simulink model "BESS_Harness"  (R2025b)
settings: Solver=VariableStepAuto  StartTime=0.0  StopTime=5  RelTol=1e-3
PostLoadFcn:
  | BESSParam
values from neighbouring files (symbols this model uses):
  bessVoltage = 1500    [BESSGFLParam.m]    (also in BESSGFMParam.m)
  gflInverter = struct    [BESSGFLParam.m]
  gfmInverter = struct    [BESSGFMParam.m]
  Ts = 5E-5    (= 5e-05)    [BESSGFLParam.m]    (also in BESSGFMParam.m; WindFarmParam.m)
undefined symbols (not defined in the file or in its folder): bessSystem, DiscIntNeverNeededParam, solar
libraries: eeGeneralControl x26, nesl_utility x26, ee_lib x16, simulink x12, fl_lib x10, eeTransforms x7, nesl_utility_internal x4, slpidlib x2, batteryecm_lib x2, simulink_extras x1, eePowerMeasurement x1, eePwmGenerator x1
(part 3 of 4)

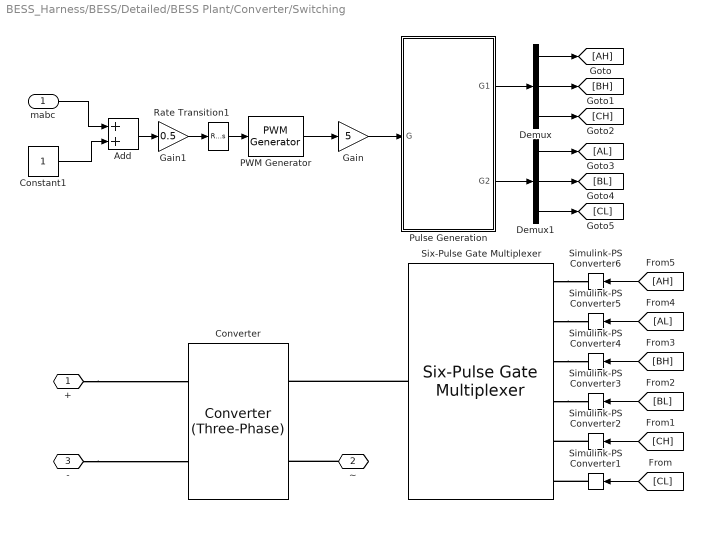
== system BESS_Harness/BESS/Detailed/BESS Plant/Converter/Switching ==
  mabc : Inport
  Add : Sum
  Constant1 : Constant
  Converter : ee_lib/Semiconductors & Converters/Converters/Converter (Three-Phase)  port_option=ee.enum.threePhasePort.composite  fidelity_option=ee.enum.converters.fidelity.detailed  device_type=ee.enum.converters.switchingdevice.ideal  showThermalPort=false  K=0  Vth=1 V  Vgt=1 V  Vgt_off=-1 V  Ih=1 A  Vf=0.8 V  Ron=0.001 Ohm  Rds=0.001 Ohm  Goff=1e-6 1/Ohm  Eon_scalar=22.86e-3 J  Eoff_scalar=17.14e-3 J  Eoff_natural_commutation=10e-3 J  Voff=300 V  Iout_scalar=600 A  onCurrentMeasDelay=0 s  useCurrentFromPreviousCycle=false  useVoltageFromPreviousCycle=false  diode_param=ee.enum.converters.protectiondiode.nodynamics  diode_Vf=0.01 V  diode_Ron=0.0001 Ohm  diode_Goff=1e-5 1/Ohm  diode_C=50 nF  diode_iRM=-235 A  diode_iF=300 A  diode_idot=-50 A/us  diode_trr_param=ee.enum.converters.diodetrr.trr_factor  diode_trr_factor=3  diode_trr=15 us  diode_Qrr=1500 s*uA  diode_rec_loss_model=ee.enum.diode.reverseRecoveryModel.fixed  diode_ErecVal=0 J  diode_scaleWithIandV=false  diode_ErecMat=zeros(2, 3) J  diode_TjrecVec=[298.15, 398.15] K  diode_IfrecVec=[.1, 1, 10] A  diode_IrecVal=10 A  diode_VrecVal=10 V  diode_tFilter=1 / 1000 / 100 s  thermal_network_parameterization=ee.enum.thermalNetworkTopology.external  Rth=[.08, .5] K/W  Rth_Cauer=[.08, .1, .5] K/W  Rth_Foster=[.08, .14, .22, .16] K/W  thermal_mass_parameterization=ee.enum.thermalNetwork.timeconstant  thermal_mass=[.01, .5] J/K  thermal_mass_Cauer=[.01, .1, .5] J/K  thermal_mass_Foster=[.001, .005, .05, .5] J/K  thermal_time_constant=[.001, .2] s  thermal_time_constant_Cauer=[.001, .1, .2] s  thermal_time_constant_Foster=[7e-05, .0007, .01, .08] s  thermal_mass_initial_temperatures=[25, 25] degC  thermal_mass_initial_temperatures_Cauer=[25, 25, 25] degC  junction_thermal_mass=0.01 J/K  Tvec_initial_Foster=[25, 25, 25, 25] degC  snubber_type=ee.enum.converters.snubber.exclude  Cs=1e-7 F  Rs=0.1 Ohm  Vce_loss=[0, 150, 300] V
  Demux : Demux  Outputs=3
  Demux1 : Demux  Outputs=3
  Gain : Gain  Gain=5
  Gain1 : Gain  Gain=0.5
  PWM Generator : eePwmGenerator/PWM Generator  CarrCount=Up  Tper=1/(fSw*1000)  Tdelay=0  Ts=1/(10*fSw*1000)
  Pulse Generation : Subsystem
  Rate Transition1 : RateTransition  OutPortSampleTime=1/(10*fSw*1000)
  Simulink-PS Converter{1..6} (6 alike) : nesl_utility/Simulink-PS Converter  PhysicalDomain=network_engine_domain  SubClassName=ps_input  LeftPortType=input  RightPortType=output  PseudoPeriodic=off  Frequencies=[]  NoiseDistribution=none  NoiseParameters=[]  Unit=1  AffineConversion=off  FilteringAndDerivatives=provide  SimscapeFilterOrder=1  InputFilterTimeConstant=0.001  UdotUserProvided=0
  Six-Pulse Gate Multiplexer : ee_lib/Semiconductors & Converters/Converters/Six-Pulse Gate Multiplexer  port_option=ee.enum.controlport.ps
  + : PMIOPort  Side=Left
  ~ : PMIOPort  Port=2  Side=Right
  - : PMIOPort  Port=3  Side=Left
  wires:
  Demux1/1 -> [AL]
  [BL] -> Simulink-PS Converter3/1
  [AH] -> Simulink-PS Converter6/1
  Demux1/3 -> [CL]
  Gain1/1 -> Rate Transition1/1
  Demux/3 -> [CH]
  Demux/2 -> [BH]
  [CL] -> Simulink-PS Converter1/1
  Constant1/1 -> Add/2
  Add/1 -> Gain1/1
  Gain/1 -> Pulse Generation/1(G)
  PWM Generator/1 -> Gain/1
  mabc/1 -> Add/1
  [CH] -> Simulink-PS Converter2/1
  [AL] -> Simulink-PS Converter5/1
  Demux1/2 -> [BL]
  Demux/1 -> [AH]
  Rate Transition1/1 -> PWM Generator/1
  Pulse Generation/2(G2) -> Demux1/1
  Pulse Generation/1(G1) -> Demux/1
  [BH] -> Simulink-PS Converter4/1
  connections:
  ~/RConn1 -- Converter/LConn2
  Six-Pulse Gate Multiplexer/LConn2 -- Simulink-PS Converter5/RConn1
  Simulink-PS Converter2/RConn1 -- Six-Pulse Gate Multiplexer/LConn5
  Simulink-PS Converter1/RConn1 -- Six-Pulse Gate Multiplexer/LConn6
  Six-Pulse Gate Multiplexer/LConn3 -- Simulink-PS Converter4/RConn1
  Six-Pulse Gate Multiplexer/RConn1 -- Converter/LConn1
  Six-Pulse Gate Multiplexer/LConn1 -- Simulink-PS Converter6/RConn1
  Six-Pulse Gate Multiplexer/LConn4 -- Simulink-PS Converter3/RConn1
  +/RConn1 -- Converter/RConn1
  -/RConn1 -- Converter/RConn2

== system BESS_Harness/BESS/Detailed/Filter & Measurements/PLL & Measurements/Measurement1 ==
  u : Inport
  Lead-Lag (Discrete or Continuous) : eeGeneralControl/Lead-Lag (Discrete or Continuous)  T1=0  T2=1e-3  B=inf  A=-inf  init_option=Inherited from block input  x0=0  Ts=Ts
  Vg : Outport
  wires:
  u/1 -> Lead-Lag (Discrete or Continuous)/1
  Lead-Lag (Discrete or Continuous)/1 -> Vg/1

== system BESS_Harness/BESS/Detailed/Filter & Measurements/PLL & Measurements/Measurement2 ==
  u : Inport
  Lead-Lag (Discrete or Continuous) : eeGeneralControl/Lead-Lag (Discrete or Continuous)  T1=0  T2=1e-3  B=inf  A=-inf  init_option=Inherited from block input  x0=0  Ts=Ts
  Vg : Outport
  wires:
  u/1 -> Lead-Lag (Discrete or Continuous)/1
  Lead-Lag (Discrete or Continuous)/1 -> Vg/1

== system BESS_Harness/BESS/Detailed/Filter & Measurements/PLL & Measurements/Subsystem ==
  Vabc : Inport
  Iabc : Inport  Port=2
  Demux : Demux  Outputs=3
  Demux1 : Demux  Outputs=3
  Park Transform : eeTransforms/Park Transform  AxisAlignment=Q-axis  PowerInvariant=off
  Park Transform1 : eeTransforms/Park Transform  AxisAlignment=Q-axis  PowerInvariant=off
  Scope : Scope  NumInputPorts=2
      settings: ActiveDisplayYMinimum=0.95416  ActiveDisplayYMaximum=1.02793  DataLoggingVariableName=ScopeData5
  Scope1 : Scope  NumInputPorts=2
      settings: ActiveDisplayYMinimum=-2.7903298017751648  ActiveDisplayYMaximum=-1.7770998587100291  DataLoggingVariableName=ScopeData10
  "Sinusoidal Measurement (PLL, Three-Phase)" : eeSinusoidalMeasurementV2/Sinusoidal Measurement (PLL, Three-Phase)  InputFilter=on  InputNormalization=off  Kp_LF=40  Ki_LF=1000  F0=frequency  Theta0=0  Ts=Ts
  Terminator : Terminator
  Terminator1 : Terminator
  mag : Outport
  freq : Outport  Port=2
  angle : Outport  Port=3
  Vd : Outport  Port=4
  Vq : Outport  Port=5
  Id1 : Outport  Port=6
  Iq1 : Outport  Port=7
  wires:
  Iabc/1 -> Park Transform1/1
  Demux1/3 -> Terminator1/1
  Demux1/2 -> Scope1/2, Iq1/1
  Demux1/1 -> Scope1/1, Id1/1
  Park Transform1/1 -> Demux1/1
  "Sinusoidal Measurement (PLL, Three-Phase)"/3 -> mag/1
  "Sinusoidal Measurement (PLL, Three-Phase)"/1 -> freq/1
  "Sinusoidal Measurement (PLL, Three-Phase)"/2 -> Park Transform/2, Park Transform1/2, angle/1
  Demux/2 -> Vq/1, Scope/2
  Demux/1 -> Vd/1, Scope/1
  Park Transform/1 -> Demux/1
  Vabc/1 -> "Sinusoidal Measurement (PLL, Three-Phase)"/1, Park Transform/1
  Demux/3 -> Terminator/1

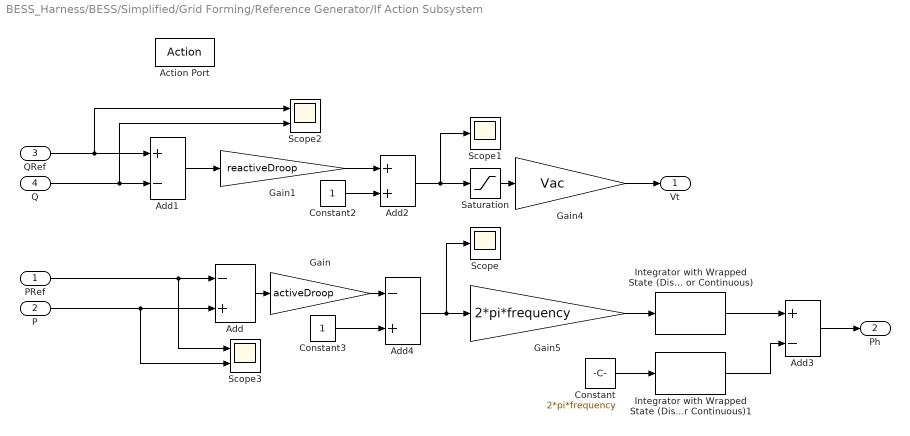
== system BESS_Harness/BESS/Simplified/Grid Forming/Reference Generator/If Action Subsystem ==
  PRef : Inport
  P : Inport  Port=2
  QRef : Inport  Port=3
  Q : Inport  Port=4
  Action Port : ActionPort  ActionPortLabel=if(u1 > 0)
  Add : Sum  Inputs=-+
  Add1 : Sum  Inputs=+-
  Add2 : Sum
  Add3 : Sum  Inputs=+-
  Add4 : Sum  Inputs=-+
  Constant : Constant  Value=2*pi*frequency  SampleTime=-1
  Constant2 : Constant
  Constant3 : Constant
  Gain : Gain  Gain=activeDroop
  Gain1 : Gain  Gain=reactiveDroop
  Gain4 : Gain  Gain=Vac
  Gain5 : Gain  Gain=2*pi*frequency
  Integrator with Wrapped State (Discrete or Continuous) : eeGeneralControl/Integrator with Wrapped State (Discrete or Continuous)  LabelModeActiveChoice=Discrete  WrappedStateUpperValue=2*pi  WrappedStateLowerValue=0  x0=0  Ts=-1
  Integrator with Wrapped State (Discrete or Continuous)1 : eeGeneralControl/Integrator with Wrapped State (Discrete or Continuous)  LabelModeActiveChoice=Discrete  WrappedStateUpperValue=2*pi  WrappedStateLowerValue=0  x0=0  Ts=-1
  Saturation : Saturate  UpperLimit=1.1  LowerLimit=0.9
  Scope : Scope
      settings: ActiveDisplayYMinimum=-1  ActiveDisplayYMaximum=1  DataLoggingVariableName=ScopeData2
  Scope1 : Scope
      settings: ActiveDisplayYMinimum=-1  ActiveDisplayYMaximum=1  DataLoggingVariableName=ScopeData3
  Scope2 : Scope  NumInputPorts=2
      settings: ActiveDisplayYMinimum=-1  ActiveDisplayYMaximum=1
  Scope3 : Scope  NumInputPorts=2
      settings: ActiveDisplayYMinimum=-1  ActiveDisplayYMaximum=1  DataLoggingVariableName=ScopeData2
  Vt : Outport
  Ph : Outport  Port=2
  wires:
  Add4/1 -> Scope/1, Gain5/1
  Gain/1 -> Add4/1
  Add1/1 -> Gain1/1
  Add2/1 -> Scope1/1, Saturation/1
  Gain5/1 -> Integrator with Wrapped State (Discrete or Continuous)/1
  Constant3/1 -> Add4/2
  Integrator with Wrapped State (Discrete or Continuous)/1 -> Add3/1
  Constant2/1 -> Add2/2
  Gain1/1 -> Add2/1
  Gain4/1 -> Vt/1
  QRef/1 -> Add1/1, Scope2/1
  Saturation/1 -> Gain4/1
  Add/1 -> Gain/1
  PRef/1 -> Add/1, Scope3/1
  Add3/1 -> Ph/1
  Constant/1 -> Integrator with Wrapped State (Discrete or Continuous)1/1
  Integrator with Wrapped State (Discrete or Continuous)1/1 -> Add3/2
  P/1 -> Add/2, Scope3/2
  Q/1 -> Add1/2, Scope2/2

== system BESS_Harness/BESS/Simplified/Grid Forming/Reference Generator/If Action Subsystem1 ==
  PRef : Inport
  P : Inport  Port=2
  VRef : Inport  Port=3
  V : Inport  Port=4
  Action Port : ActionPort  ActionPortLabel=else
  Add : Sum  Inputs=+-
  Add1 : Sum  Inputs=+-
  Add2 : Sum
  Add3 : Sum  Inputs=+-
  Add4 : Sum  Inputs=-+
  Constant2 : Constant
  Constant3 : Constant
  Constant4 : Constant  Value=0
  Gain : Gain  Gain=reactiveDroop
  Gain1 : Gain  Gain=activeDroop
  Gain4 : Gain  Gain=systemVoltage
  Gain5 : Gain  Gain=2*pi*systemFrequency
  Integrator with Wrapped State (Discrete or Continuous) : eeGeneralControl/Integrator with Wrapped State (Discrete or Continuous)  LabelModeActiveChoice=Discrete  WrappedStateUpperValue=2*pi  WrappedStateLowerValue=0  x0=0  Ts=-1
  Saturation : Saturate  UpperLimit=1.1  LowerLimit=0.9
  Vt : Outport
  Ph : Outport  Port=2
  wires:
  Add/1 -> Gain/1
  Constant4/1 -> Add3/2
  Add4/1 -> Gain5/1
  Gain/1 -> Add4/1
  Add1/1 -> Gain1/1
  Add2/1 -> Saturation/1
  Gain5/1 -> Integrator with Wrapped State (Discrete or Continuous)/1
  Constant3/1 -> Add4/2
  Integrator with Wrapped State (Discrete or Continuous)/1 -> Add3/1
  Constant2/1 -> Add2/2
  Gain1/1 -> Add2/1
  V/1 -> Add/2
  Gain4/1 -> Vt/1
  P/1 -> Add1/2
  VRef/1 -> Add/1
  PRef/1 -> Add1/1
  Add3/1 -> Ph/1
  Saturation/1 -> Gain4/1

== system BESS_Harness/BESS/Detailed/BESS Controller/Grid Following/Reference Current/Current limits ==
  Imax : Inport
  iqref : Inport  Port=2
  idref : Inport  Port=3
  Constant8 : Constant  Value=0
  Constant9 : Constant  Value=0
  Scope : Scope
      settings: ActiveDisplayYMinimum=-0.14399  ActiveDisplayYMaximum=1.29587  DataLoggingVariableName=ScopeData3
  Scope1 : Scope
      settings: ActiveDisplayYMinimum=-0.13655  ActiveDisplayYMaximum=1.22893  DataLoggingVariableName=ScopeData4
  Sqrt : Sqrt
  Sqrt1 : Sqrt
  Square{1..4} (4 alike) : Math  Operator=square
  Step2 : Step  Time=0.01  SampleTime=Ts
  Step3 : Step  Time=0.01  SampleTime=Ts
  Sum6 : Sum  Inputs=|+-
  Sum9 : Sum  Inputs=|+-
  Switch1 : Switch  Threshold=.01  SaturateOnIntegerOverflow=off  InputSameDT=off
  Switch2 : Switch  Threshold=.01  SaturateOnIntegerOverflow=off  InputSameDT=off
  iubq : Outport
  iubd : Outport  Port=2
  wires:
  idref/1 -> Square4/1
  Sqrt1/1 -> iubq/1, Scope1/1
  Imax/1 -> Square1/1, Square3/1
  Sqrt/1 -> iubd/1, Scope/1
  Constant9/1 -> Switch2/3
  Square4/1 -> Sum9/2
  Constant8/1 -> Switch1/3
  Square2/1 -> Sum6/2
  Sum6/1 -> Switch1/1
  Square3/1 -> Sum9/1
  iqref/1 -> Square2/1
  Switch1/1 -> Sqrt/1
  Square1/1 -> Sum6/1
  Switch2/1 -> Sqrt1/1
  Step2/1 -> Switch1/2
  Step3/1 -> Switch2/2
  Sum9/1 -> Switch2/1

== system BESS_Harness/BESS/Detailed/BESS Controller/Grid Following/Reference Current/Refernce id generation ==
  V_mag : Inport
  del f : Inport  Port=2
  ubid : Inport  Port=3
  PRef : Inport  Port=4
  Divide : Product  Inputs=/*
  Gain6 : Gain  Gain=-1
  P/Q Priority : Switch  Criteria=u2 ~= 0  SaturateOnIntegerOverflow=off  InputSameDT=off
  Priority Mode : Constant  Value=P-2
  Saturation Dynamic2 : simulink/Discontinuities/Saturation Dynamic  OutMin=[]  OutMax=[]  OutDataTypeStr=Inherit: Same as second input  OutDataType=fixdt(1, 16)  OutScaling=2^-10  DoSatur=off
  Saturation1 : Saturate  UpperLimit=Imax  LowerLimit=-Imax
  Scope : Scope
      settings: ActiveDisplayYMinimum=-1  ActiveDisplayYMaximum=1
  Scope1 : Scope
      settings: ActiveDisplayYMinimum=-0.68622  ActiveDisplayYMaximum=0.07625  DataLoggingVariableName=ScopeData2
  Sum : Sum  Inputs=|++
  droop m_p : Gain  Gain=mp/MVA
  ubid1 : InportShadow  Port=3
  id_ref : Outport
  wires:
  del f/1 -> droop m_p/1
  Divide/1 -> Saturation Dynamic2/2, Saturation1/1
  V_mag/1 -> Divide/1
  P/Q Priority/1 -> id_ref/1, Scope/1
  ubid1/1 -> Gain6/1
  Saturation1/1 -> P/Q Priority/1
  Priority Mode/1 -> P/Q Priority/2
  PRef/1 -> Sum/2
  Saturation Dynamic2/1 -> P/Q Priority/3, Scope1/1
  Gain6/1 -> Saturation Dynamic2/3
  ubid/1 -> Saturation Dynamic2/1
  Sum/1 -> Divide/2
  droop m_p/1 -> Sum/1

== system BESS_Harness/BESS/Detailed/BESS Controller/Grid Following/Reference Current/Refernce iq generation ==
  ubiq : Inport
  V_ref : Inport  Port=2
  V_mag : Inport  Port=3
  LVRT_iq : Inport  Port=4
  Q_ref : Inport  Port=5
  Divide1 : Product  Inputs=*/
  Gain : Gain  Gain=-1
  Gain1 : Gain  Gain=-1
  Gain7 : Gain  Gain=-1
  LVRT Priority : Switch  Threshold=.9  SaturateOnIntegerOverflow=off  InputSameDT=off
  P/Q Priority : Switch  Criteria=u2 ~= 0  SaturateOnIntegerOverflow=off  InputSameDT=off
  Priority Mode : Constant  Value=P-2
  Saturation Dynamic : simulink/Discontinuities/Saturation Dynamic  OutMin=[]  OutMax=[]  OutDataTypeStr=Inherit: Same as second input  OutDataType=fixdt(1, 16)  OutScaling=2^-10  DoSatur=off
  Saturation2 : Saturate  UpperLimit=1  LowerLimit=-1
  Saturation3 : Saturate  UpperLimit=Imax  LowerLimit=-Imax
  Sum : Sum  Inputs=|++
  Sum1 : Sum  Inputs=|-+
  droop m_v : Gain  Gain=mv
  ubiq1 : InportShadow
  iq_ref : Outport
  wires:
  Gain/1 -> iq_ref/1
  V_mag/1 -> Sum1/2, Divide1/2, LVRT Priority/2
  Q_ref/1 -> Sum/1
  Sum/1 -> Divide1/1
  droop m_v/1 -> Sum/2
  ubiq1/1 -> Gain7/1
  LVRT_iq/1 -> Saturation2/1
  V_ref/1 -> Sum1/1
  Gain7/1 -> Saturation Dynamic/3
  Saturation Dynamic/1 -> P/Q Priority/1
  Divide1/1 -> Saturation3/1, Saturation Dynamic/2
  Priority Mode/1 -> P/Q Priority/2
  Saturation3/1 -> P/Q Priority/3
  Saturation2/1 -> Gain1/1
  ubiq/1 -> Saturation Dynamic/1
  Gain1/1 -> LVRT Priority/3
  P/Q Priority/1 -> LVRT Priority/1
  Sum1/1 -> droop m_v/1
  LVRT Priority/1 -> Gain/1

== system BESS_Harness/BESS/Detailed/BESS Controller/Grid Forming/Current Limiting/CurrentLimitingMethod ==
  Igd : Inport
  Igq : Inport  Port=2
  currentLimitAndVirtual : Subsystem  VariantControl=both
  currentSaturation : Subsystem  VariantControl=ctSat
  virtualImpedance : Subsystem  VariantControl=virimp
  delVd : Outport
  delVq : Outport  Port=2
  Idmax : Outport  Port=3
  Iqmax : Outport  Port=4

== system BESS_Harness/BESS/Detailed/BESS Controller/Grid Forming/Grid Voltage Reactive Power Support/Modifying Active Power Reference ==
  PrefInput : Inport
  Vd : Inport  Port=2
  Igd : Inport  Port=3
  Igq : Inport  Port=4
  AND : Logic  IconShape=distinctive  AllPortsSameDT=off  OutDataTypeStr=boolean
  Abs : Abs  SaturateOnIntegerOverflow=off
  Compare To Constant : simulink/Logic and Bit Operations/Compare To Constant  relop=>=  const=0.95  OutDataTypeStr=boolean
  Computing New Active Power Ref : Subsystem
  Math Function1 : Math  Operator=hypot
  Power Sign : Signum
  Product : Product
  Relay : Relay  OnSwitchValue=40%maxVICurrentLimit*0.96  OffSwitchValue=1
  Scope : Scope
  Scope1 : Scope
  Scope2 : Scope
  Switch : Switch  Criteria=u2 > Threshold  SaturateOnIntegerOverflow=off  InputSameDT=off
  Pref : Outport
  wires:
  Compare To Constant/1 -> AND/1
  AND/1 -> Switch/2
  Relay/1 -> AND/2, Scope1/1
  Product/1 -> Pref/1
  Power Sign/1 -> Product/2
  Abs/1 -> Product/1
  Switch/1 -> Abs/1
  Igq/1 -> Math Function1/1, Computing New Active Power Ref/1(Iq)
  Igd/1 -> Math Function1/2
  PrefInput/1 -> Switch/3, Power Sign/1
  Vd/1 -> Compare To Constant/1, Computing New Active Power Ref/2(Vd)
  Math Function1/1 -> Relay/1, Scope2/1  "Is"
  Computing New Active Power Ref/1(Pref) -> Scope/1, Switch/1

== system BESS_Harness/BESS/Detailed/BESS Controller/Grid Forming/Grid Voltage Reactive Power Support/Modifying Reactive Power Reference ==
  Vgd : Inport
  Vgq : Inport  Port=2
  Qref : Inport  Port=3
  Pref : Inport  Port=4
  Changing the Power Reference : Subsystem
  Hysteresis : Subsystem
  Math Function : Math  Operator=hypot
  Merge : Merge
  Merge1 : Merge
  NOT : Logic  Operator=NOT  IconShape=distinctive  AllPortsSameDT=off  OutDataTypeStr=boolean
  Not Altering the Power Reference : Subsystem
  Scope : Scope
  PrefNew : Outport
  QrefNew : Outport  Port=2
  wires:
  [Qref] -> Changing the Power Reference/4(Qref)
  [Pref] -> Changing the Power Reference/3(Pref)
  Merge/1 -> PrefNew/1
  Merge1/1 -> QrefNew/1
  Pref/1 -> [Pref], Not Altering the Power Reference/1(Pref)
  Vgq/1 -> Math Function/2
  Changing the Power Reference/2(Qrefv) -> Merge1/1
  [Vd] -> Changing the Power Reference/2(Vd)
  Hysteresis/1(LVFlag) -> NOT/1, Changing the Power Reference/Enable, Scope/1
  Qref/1 -> [Qref], Not Altering the Power Reference/2(Qref)
  NOT/1 -> Not Altering the Power Reference/Enable
  Changing the Power Reference/1(Prefv) -> Merge/1
  Not Altering the Power Reference/1(Prefv) -> Merge/2
  [Vs] -> Changing the Power Reference/1(Vs)
  Math Function/1 -> [Vs], Hysteresis/1(Vs)
  Not Altering the Power Reference/2(Qrefv) -> Merge1/2
  Vgd/1 -> Math Function/1, [Vd]

== system BESS_Harness/BESS/Detailed/BESS Controller/Grid Forming/Measurement/Frequency Measurement ==
  Vabc : Inport
  Convert To PU : Gain  Gain=1/powerFreq
  Frequency Measurement : Subsystem  TreatAsAtomicUnit=on  SystemSampleTime=sampleTime  mask{initialFrequency=powerFreq, sampleTime=activePowerSampleTime}
      mask prompts: initialFrequency "Initial frequency in Hz"; sampleTime "Sample time in sec"
      mask DialogControl Container7 Prompt: General
  Low-Pass Filter : eeGeneralControl/Low-Pass Filter (Discrete or Continuous)  K=1  T=freqMeasTimeConst  B=inf  A=-inf  init_option=Inherited from block input  x0=0  Ts=-1
  freq : Outport
  wires:
  Vabc/1 -> Frequency Measurement/1(abc)
  Convert To PU/1 -> freq/1
  Frequency Measurement/1(Freq) -> Low-Pass Filter/1
  Low-Pass Filter/1 -> Convert To PU/1  "Freq"

== system BESS_Harness/BESS/Detailed/BESS Controller/Grid Forming/Measurement/abc2dq ==
  Igabc : Inport
  Angle : Inport  Port=2
  Vgabc : Inport  Port=3
  Supply Current to dq : Subsystem
  Supply Voltage  to dq1 : Subsystem
  Vgd : Outport
  Vgq : Outport  Port=2
  Igd : Outport  Port=3
  Igq : Outport  Port=4
  wires:
  Supply Voltage  to dq1/2(Vgq) -> Vgq/1  "Vgq"
  Supply Voltage  to dq1/1(Vgd) -> Vgd/1  "Vgd"
  Supply Current to dq/2(Igq) -> Igq/1  "Iq"
  Supply Current to dq/1(Igd) -> Igd/1  "Id"
  Igabc/1 -> Supply Current to dq/1(abc)
  Vgabc/1 -> Supply Voltage  to dq1/2(abc)
  Angle/1 -> Supply Current to dq/2(Angle), Supply Voltage  to dq1/1(Angle)

== system BESS_Harness/BESS/Detailed/BESS Controller/Grid Forming/Power Control/ActivePowerControl ==
  Pref : Inport
  Pmeas : Inport  Port=2
  fref : Inport  Port=3
  cntrlflag : Inport  Port=4
  fgrid : Inport  Port=5
  droopControl : Subsystem  VariantControl=droop
  vsmControl : Subsystem  VariantControl=vsm
  Theta : Outport
  w : Outport  Port=2

== system BESS_Harness/BESS/Detailed/BESS Controller/Grid Forming/Power Control/ReactiveControl ==
  note: Vs-delV
  CntrlFlag : Inport
  Qref : Inport  Port=2
  Qmeas : Inport  Port=3
  Vgdmeas : Inport  Port=4
  Vref : Inport  Port=5
  Constant2 : Constant  Value=0
  Saturation1 : Saturate  UpperLimit=(dcBusVoltage/2)/(sqrt(2/3)*girdLineVoltage)  LowerLimit=-(dcBusVoltage/2)/(sqrt(2/3)*girdLineVoltage)
  Scope : Scope
      settings: ActiveDisplayYMinimum=0.99958  ActiveDisplayYMaximum=1.0007  DataLoggingVariableName=ScopeData20
  Voltage  Reference Selection : Subsystem
  Vmd : Outport
  Vmq : Outport  Port=2
  wires:
  Vgdmeas/1 -> Voltage  Reference Selection/5(Vgdmeas)
  Vref/1 -> Voltage  Reference Selection/4(Vref)
  Qmeas/1 -> Voltage  Reference Selection/3(Qmeas)
  Qref/1 -> Voltage  Reference Selection/2(Qref)
  CntrlFlag/1 -> Voltage  Reference Selection/1(cntrlflag)
  Saturation1/1 -> Vmd/1, Scope/1
  Constant2/1 -> Vmq/1
  Voltage  Reference Selection/1(Vd) -> Saturation1/1  "Q"

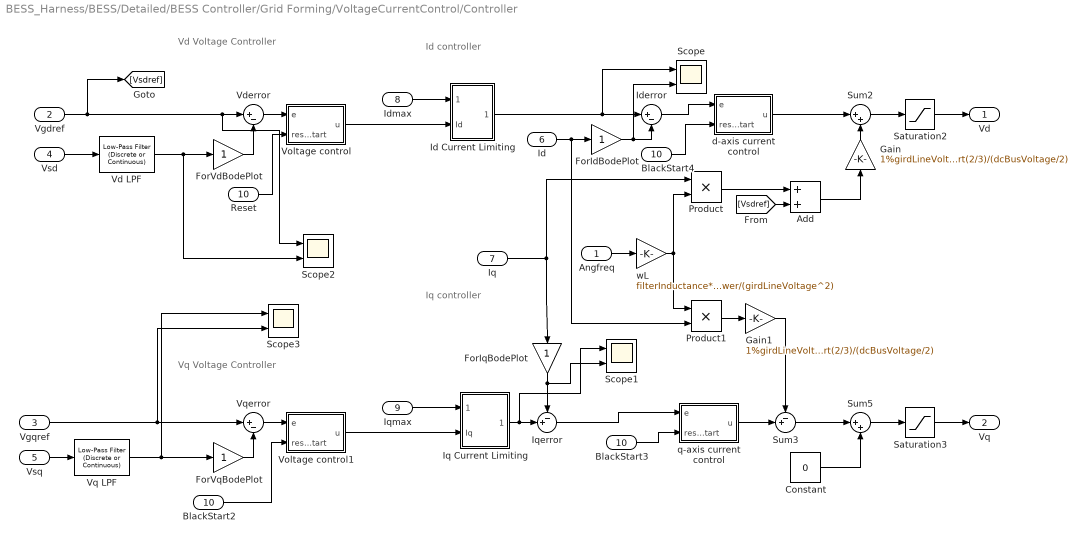
== system BESS_Harness/BESS/Detailed/BESS Controller/Grid Forming/VoltageCurrentControl/Controller ==
  note: Vq Voltage Controller
  note: Iq controller
  note: Vd Voltage Controller
  note: Id controller
  Angfreq : Inport
  Vgdref : Inport  Port=2
  Vgqref : Inport  Port=3
  Vsd : Inport  Port=4
  Vsq : Inport  Port=5
  Id : Inport  Port=6
  Iq : Inport  Port=7
  Idmax : Inport  Port=8
  Iqmax : Inport  Port=9
  Reset : Inport  Port=10
  Add : Sum
  BlackStart2 : InportShadow  Port=10
  BlackStart3 : InportShadow  Port=10
  BlackStart4 : InportShadow  Port=10
  Constant : Constant  Value=0  SampleTime=currentControlTs
  ForIdBodePlot : Gain
  ForIqBodePlot : Gain
  ForVdBodePlot : Gain
  ForVqBodePlot : Gain
  Gain : Gain  Gain=1%girdLineVoltage*sqrt(2/3)/(dcBusVoltage/2)
  Gain1 : Gain  Gain=1%girdLineVoltage*sqrt(2/3)/(dcBusVoltage/2)
  Id Current Limiting : Subsystem
  Iderror : Sum  Inputs=|+-
  Iq Current Limiting : Subsystem
  Iqerror : Sum  Inputs=-+|
  Product : Product
  Product1 : Product
  Saturation2 : Saturate  UpperLimit=4  LowerLimit=-3
  Saturation3 : Saturate  UpperLimit=3  LowerLimit=-3
  Scope{,1..3} (4 alike) : Scope  NumInputPorts=2
      Scope settings: ActiveDisplayYMinimum=-0.33488  ActiveDisplayYMaximum=2.03721
      Scope2 settings: ActiveDisplayYMinimum=-0.14129  ActiveDisplayYMaximum=1.2716
  Sum2 : Sum  Inputs=|++
  Sum3 : Sum  Inputs=-+|
  Sum5 : Sum  Inputs=|++
  Vd LPF : eeGeneralControl/Low-Pass Filter (Discrete or Continuous)  K=1  T=vdvqLPFTimeConst  B=inf  A=-inf  init_option=Specify as parameter  x0=0  Ts=voltControlTs
  Vderror : Sum  Inputs=|+-
  Voltage control : Subsystem
  Voltage control1 : Subsystem
  Vq LPF : eeGeneralControl/Low-Pass Filter (Discrete or Continuous)  K=1  T=vdvqLPFTimeConst  B=inf  A=-inf  init_option=Inherited from block input  x0=0  Ts=voltControlTs
  Vqerror : Sum  Inputs=|+-
  d-axis current control : Subsystem
  q-axis current control : Subsystem
  wL : Gain  Gain=filterInductance*power/(girdLineVoltage^2)
  Vd : Outport  VectorParamsAs1DForOutWhenUnconnected=off
  Vq : Outport  Port=2  VectorParamsAs1DForOutWhenUnconnected=off
  wires:
  Vgdref/1 -> [Vsdref], Vderror/1, Scope2/1
  BlackStart4/1 -> d-axis current control/2(resetBlackStart)
  BlackStart3/1 -> q-axis current control/2(resetBlackStart)
  BlackStart2/1 -> Voltage control1/2(resetBlackStart)
  Reset/1 -> Voltage control/2(resetBlackStart)
  Vq LPF/1 -> ForVqBodePlot/1, Scope3/1
  Vd LPF/1 -> ForVdBodePlot/1, Scope2/2
  Id Current Limiting/1(Idref) -> Iderror/1, Scope/1
  ForIqBodePlot/1 -> Iqerror/1, Scope1/2
  ForIdBodePlot/1 -> Iderror/2, Scope/2
  ForVqBodePlot/1 -> Vqerror/2
  ForVdBodePlot/1 -> Vderror/2
  Vsd/1 -> Vd LPF/1
  Voltage control1/1(u) -> Iq Current Limiting/2(Iq)
  Iq Current Limiting/1(Iqref) -> Iqerror/2, Scope1/1
  Idmax/1 -> Id Current Limiting/1(Imax)
  Voltage control/1(u) -> Id Current Limiting/2(Id)
  Gain/1 -> Sum2/2
  Add/1 -> Gain/1
  [Vsdref] -> Add/2
  Gain1/1 -> Sum3/1
  Vqerror/1 -> Voltage control1/1(e)
  Vgqref/1 -> Vqerror/1, Scope3/2
  Iqmax/1 -> Iq Current Limiting/1(Imax)
  Vderror/1 -> Voltage control/1(e)
  Id/1 -> ForIdBodePlot/1, Product1/2
  Vsq/1 -> Vq LPF/1
  Sum5/1 -> Saturation3/1
  Sum3/1 -> Sum5/1
  q-axis current control/1(u) -> Sum3/2
  Sum2/1 -> Saturation2/1
  d-axis current control/1(u) -> Sum2/1
  Product/1 -> Add/1
  Product1/1 -> Gain1/1
  Saturation2/1 -> Vd/1
  Saturation3/1 -> Vq/1
  Iderror/1 -> d-axis current control/1(e)
  Constant/1 -> Sum5/2
  Angfreq/1 -> wL/1
  Iq/1 -> Product/1, ForIqBodePlot/1
  wL/1 -> Product/2, Product1/1
  Iqerror/1 -> q-axis current control/1(e)

== system BESS_Harness/BESS/Detailed/BESS Controller/Grid Forming/VoltageCurrentControl/Modulation Signal ==
  Vd : Inport
  Vq : Inport  Port=2
  Angle : Inport  Port=3
  Constant : Constant  Value=0
  Inverse Park Transform : eeTransforms/Inverse Park Transform  AxisAlignment=D-axis  PowerInvariant=off
  Mux1 : Mux  Inputs=3
  Saturation2 : Saturate  UpperLimit=1  LowerLimit=-1
  Scope : Scope  NumInputPorts=2
      settings: DataLoggingVariableName=ScopeData9
  Scope1 : Scope
  mabc : Outport  VectorParamsAs1DForOutWhenUnconnected=off
  wires:
  Vq/1 -> Mux1/2, Scope/2
  Vd/1 -> Mux1/1, Scope/1
  Constant/1 -> Mux1/3
  Saturation2/1 -> mabc/1
  Angle/1 -> Inverse Park Transform/2, Scope1/1
  Mux1/1 -> Inverse Park Transform/1
  Inverse Park Transform/1 -> Saturation2/1

== system BESS_Harness/BESS/Detailed/BESS Plant/Converter/Switching/Pulse Generation ==
  G : Inport
  Constant : Constant  Value=5
  Subtract : Sum  Inputs=-+
  G1 : Outport  VectorParamsAs1DForOutWhenUnconnected=off
  G2 : Outport  Port=2  VectorParamsAs1DForOutWhenUnconnected=off
  wires:
  G/1 -> Subtract/1, G1/1
  Constant/1 -> Subtract/2
  Subtract/1 -> G2/1

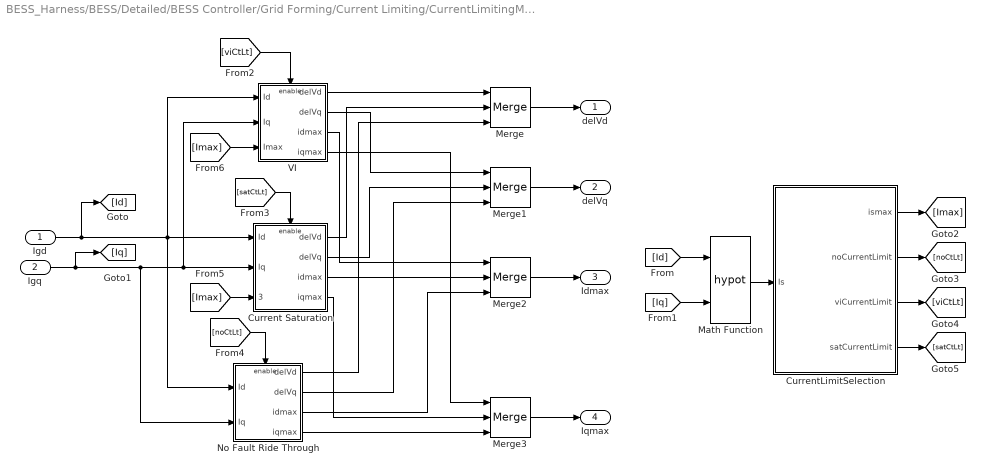
== system BESS_Harness/BESS/Detailed/BESS Controller/Grid Forming/Current Limiting/CurrentLimitingMethod/currentLimitAndVirtual ==
  Igd : Inport
  Igq : Inport  Port=2
  Current Saturation : Subsystem
  CurrentLimitSelection : Stateflow chart  TreatAsAtomicUnit=on
  Math Function : Math  Operator=hypot
  Merge{,1..3} (4 alike) : Merge  Inputs=3
  No Fault Ride Through : Subsystem
  VI : Subsystem
  delVd : Outport
  delVq : Outport  Port=2
  Idmax : Outport  Port=3
  Iqmax : Outport  Port=4
  wires:
  [Imax] -> VI/3(Imax)
  [Imax] -> Current Saturation/3(Imaxsat)
  [noCtLt] -> No Fault Ride Through/Enable
  [satCtLt] -> Current Saturation/Enable
  [viCtLt] -> VI/Enable
  CurrentLimitSelection/4(satCurrentLimit) -> [satCtLt]
  CurrentLimitSelection/3(viCurrentLimit) -> [viCtLt]
  CurrentLimitSelection/2(noCurrentLimit) -> [noCtLt]
  CurrentLimitSelection/1(ismax) -> [Imax]
  Math Function/1 -> CurrentLimitSelection/1(Is)
  No Fault Ride Through/2(delVq) -> Merge1/3
  Merge3/1 -> Iqmax/1
  Current Saturation/2(delVq) -> Merge1/2
  No Fault Ride Through/4(iqmax) -> Merge3/3
  VI/3(idmax) -> Merge2/1
  VI/4(iqmax) -> Merge3/1
  Current Saturation/3(idmax) -> Merge2/2
  VI/2(delVq) -> Merge1/1
  Merge/1 -> delVd/1
  Current Saturation/4(iqmax) -> Merge3/2
  Current Saturation/1(delVd) -> Merge/2
  [Id] -> Math Function/1
  [Iq] -> Math Function/2
  VI/1(delVd) -> Merge/1
  No Fault Ride Through/3(idmax) -> Merge2/3
  No Fault Ride Through/1(delVd) -> Merge/3
  Igd/1 -> [Id], No Fault Ride Through/1(Id), Current Saturation/1(Id), VI/1(Id)
  Merge1/1 -> delVq/1
  Igq/1 -> [Iq], No Fault Ride Through/2(Iq), VI/2(Iq), Current Saturation/2(Iq)
  Merge2/1 -> Idmax/1

== system BESS_Harness/BESS/Detailed/BESS Controller/Grid Forming/Current Limiting/CurrentLimitingMethod/currentSaturation ==
  note: Vs-delV
  Igd : Inport
  Igq : Inport  Port=2
  Compare : Subsystem
  Constant : Constant  Value=maxSatCurrentLimit
  Constant1 : Constant  Value=0
  Constant2 : Constant  Value=0
  If : If
  If Action Subsystem : Subsystem  TreatAsAtomicUnit=on
  If Action Subsystem1 : Subsystem  TreatAsAtomicUnit=on
  Math Function : Math  Operator=hypot
  Merge : Merge
  Merge1 : Merge
  Subtract : Sum  Inputs=+-
  delVd : Outport
  delVq : Outport  Port=2
  Idmax : Outport  Port=3
  Iqmax : Outport  Port=4
  wires:
  Merge1/1 -> Iqmax/1
  Merge/1 -> Idmax/1
  Constant1/1 -> delVd/1
  Constant2/1 -> delVq/1
  If Action Subsystem1/2(Iqmax) -> Merge1/2
  If Action Subsystem/2(Iqmax) -> Merge1/1
  If Action Subsystem1/1(Idmax) -> Merge/2
  If Action Subsystem/1(Idmax) -> Merge/1
  [Is] -> If Action Subsystem/1(Is)
  If/2 -> If Action Subsystem1/Action
  Compare/1(Out1) -> If/1
  Subtract/1 -> Compare/1(u)
  [Isq] -> If Action Subsystem/3(Isq)
  [Isd] -> If Action Subsystem/2(Isd)
  If/1 -> If Action Subsystem/Action
  Math Function/1 -> Subtract/2, [Is]  "Is"
  Constant/1 -> Subtract/1
  Igq/1 -> Math Function/2, [Isq]
  Igd/1 -> Math Function/1, [Isd]

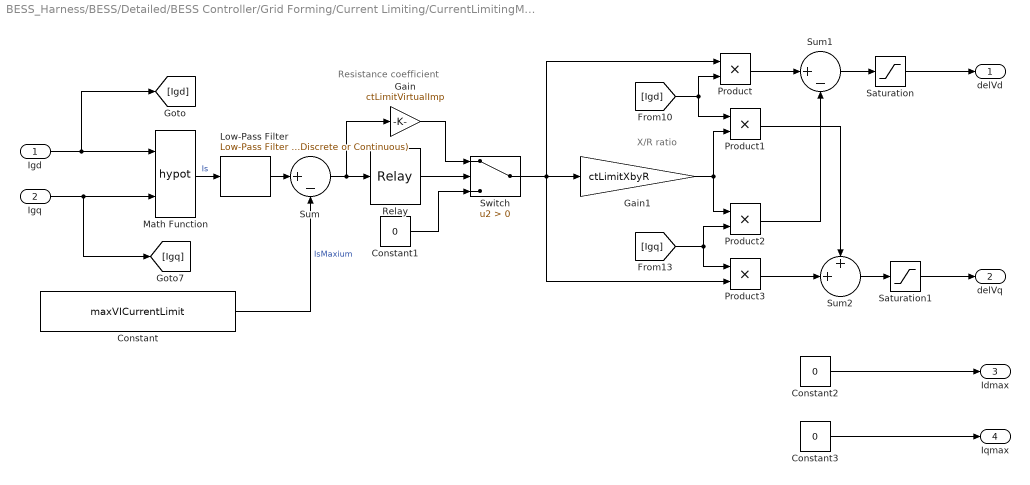
== system BESS_Harness/BESS/Detailed/BESS Controller/Grid Forming/Current Limiting/CurrentLimitingMethod/virtualImpedance ==
  note: Resistance coefficient
  note: X/R ratio
  Igd : Inport
  Igq : Inport  Port=2
  Constant : Constant  Value=maxVICurrentLimit
  Constant1 : Constant  Value=0
  Constant2 : Constant  Value=0
  Constant3 : Constant  Value=0
  Gain : Gain  Gain=ctLimitVirtualImp
  Gain1 : Gain  Gain=ctLimitXbyR
  Low-Pass Filter : eeGeneralControl/Low-Pass Filter (Discrete or Continuous)  K=1  T=currentVITimeConst  B=inf  A=-inf  init_option=Inherited from block input  x0=0  Ts=-1
  Math Function : Math  Operator=hypot
  Product{,1..3} (4 alike) : Product
  Relay : Relay  OnSwitchValue=0.01  OffSwitchValue=-0.05
  Saturation : Saturate  UpperLimit=1  LowerLimit=-1
  Saturation1 : Saturate  UpperLimit=1  LowerLimit=-1
  Sum : Sum  Inputs=|+-
  Sum1 : Sum  Inputs=|+-
  Sum2 : Sum  Inputs=++|
  Switch : Switch  Criteria=u2 > Threshold  SaturateOnIntegerOverflow=off  InputSameDT=off
  delVd : Outport
  delVq : Outport  Port=2
  Idmax : Outport  Port=3
  Iqmax : Outport  Port=4
  wires:
  Sum2/1 -> Saturation1/1
  Product3/1 -> Sum2/2
  Low-Pass Filter/1 -> Sum/1
  Saturation/1 -> delVd/1
  Relay/1 -> Switch/2
  Saturation1/1 -> delVq/1
  Igd/1 -> [Igd], Math Function/1
  Constant1/1 -> Switch/3
  Gain/1 -> Switch/1
  Constant3/1 -> Iqmax/1
  Constant2/1 -> Idmax/1
  [Igd] -> Product/2, Product1/1
  Switch/1 -> Product/1, Product3/2, Gain1/1
  [Igq] -> Product2/2, Product3/1
  Math Function/1 -> Low-Pass Filter/1  "Is"
  Constant/1 -> Sum/2  "IsMaxium"
  Product2/1 -> Sum1/2
  Product/1 -> Sum1/1
  Sum1/1 -> Saturation/1
  Gain1/1 -> Product2/1, Product1/2
  Product1/1 -> Sum2/1
  Igq/1 -> Math Function/2, [Igq]
  Sum/1 -> Relay/1, Gain/1

== system BESS_Harness/BESS/Detailed/BESS Controller/Grid Forming/Grid Voltage Reactive Power Support/Modifying Active Power Reference/Computing New Active Power Ref ==
  Iq : Inport
  Vd : Inport  Port=2
  Abs : Abs  SaturateOnIntegerOverflow=off
  Constant : Constant  Value=maxVICurrentLimit*0.96
  Constant1 : Constant  Value=0
  Product : Product
  Sqrt : Sqrt
  Square : Math  Operator=square
  Square1 : Math  Operator=square
  Subtract : Sum  Inputs=-+
  Switch : Switch  Criteria=u2 > Threshold  Threshold=1.15  SaturateOnIntegerOverflow=off  InputSameDT=off
  Pref : Outport
  wires:
  Product/1 -> Pref/1
  Iq/1 -> Square/1
  Sqrt/1 -> Abs/1
  Vd/1 -> Product/1
  Constant1/1 -> Switch/1
  Square1/1 -> Subtract/2
  Square/1 -> Switch/2, Subtract/1
  Switch/1 -> Product/2
  Subtract/1 -> Sqrt/1
  Constant/1 -> Square1/1
  Abs/1 -> Switch/3

== system BESS_Harness/BESS/Detailed/BESS Controller/Grid Forming/Grid Voltage Reactive Power Support/Modifying Reactive Power Reference/Changing the Power Reference ==
  Vs : Inport
  Vd : Inport  Port=2
  Pref : Inport  Port=3
  Qref : Inport  Port=4
  Enable : EnablePort
  ActivePowerReference : Subsystem
  Constant1 : Constant  Value=voltreference*0.96
  EstimateIdForGivenIq : Subsystem
  EstimateIqForReactivePower : Subsystem
  Max : MinMax  Function=max  Inputs=2
  ReactivePowerReference : Subsystem
  Prefv : Outport
  Qrefv : Outport  Port=2
  wires:
  Vd/1 -> EstimateIqForReactivePower/2(Vd)
  Qref/1 -> Max/2
  ReactivePowerReference/1(QrefNew) -> Max/1
  Pref/1 -> ActivePowerReference/3(Pref)
  EstimateIdForGivenIq/1(Id) -> ActivePowerReference/1(Id)
  Vs/1 -> ReactivePowerReference/1(Vd), EstimateIqForReactivePower/3(Vs), ActivePowerReference/2(Vd)
  Constant1/1 -> EstimateIqForReactivePower/1(Vmin)
  EstimateIqForReactivePower/1(Iq) -> ReactivePowerReference/2(Iq), EstimateIdForGivenIq/1(Iq)
  Max/1 -> Qrefv/1
  ActivePowerReference/1(PrefNew) -> Prefv/1

== system BESS_Harness/BESS/Detailed/BESS Controller/Grid Forming/Grid Voltage Reactive Power Support/Modifying Reactive Power Reference/Hysteresis ==
  Vs : Inport
  AND : Logic  IconShape=distinctive  AllPortsSameDT=off  OutDataTypeStr=boolean
  Compare To Constant : simulink/Logic and Bit Operations/Compare To Constant  relop=<  const=0.9  OutDataTypeStr=boolean
  Compare To Constant1 : simulink/Logic and Bit Operations/Compare To Constant  relop=<  const=0.95  OutDataTypeStr=boolean
  D Latch : simulink_extras/Flip Flops/D Latch
  OR : Logic  Operator=OR  IconShape=distinctive  AllPortsSameDT=off  OutDataTypeStr=boolean
  Scope : Scope
      settings: ActiveDisplayYMinimum=0.96929  ActiveDisplayYMaximum=1.01111
  Terminator : Terminator
  LVFlag : Outport
  wires:
  Vs/1 -> Compare To Constant/1, Compare To Constant1/1, Scope/1
  Compare To Constant/1 -> OR/2, D Latch/2, D Latch/1
  D Latch/2 -> Terminator/1
  OR/1 -> LVFlag/1
  AND/1 -> OR/1
  D Latch/1 -> AND/2
  Compare To Constant1/1 -> AND/1

== system BESS_Harness/BESS/Detailed/BESS Controller/Grid Forming/Grid Voltage Reactive Power Support/Modifying Reactive Power Reference/Not Altering the Power Reference ==
  Pref : Inport
  Qref : Inport  Port=2
  Enable : EnablePort
  Prefv : Outport
  Qrefv : Outport  Port=2
  wires:
  Qref/1 -> Qrefv/1
  Pref/1 -> Prefv/1

== system BESS_Harness/BESS/Detailed/BESS Controller/Grid Forming/Measurement/Frequency Measurement/Frequency Measurement ==
  abc : Inport
  Constant : Constant
  Discrete-Time Integrator : DiscreteIntegrator  SampleTime=sampleTime  LimitOutput=on  ICPrevOutput=DiscIntNeverNeededParam  ICPrevScaledInput=DiscIntNeverNeededParam
  If : If  IfExpression=u1 > 0.9
  If Action Subsystem : Subsystem  TreatAsAtomicUnit=on
  If Action Subsystem1 : Subsystem  TreatAsAtomicUnit=on
  Merge : Merge
  Postive Sequence : Subsystem
  Freq : Outport
  wires:
  Postive Sequence/1(posSeq) -> If Action Subsystem/1(V)
  Merge/1 -> Freq/1
  If Action Subsystem1/1(Out1) -> Merge/2
  If Action Subsystem/1(Freq) -> Merge/1
  Constant/1 -> Discrete-Time Integrator/1
  abc/1 -> Postive Sequence/1(abc)
  Discrete-Time Integrator/1 -> If/1, If Action Subsystem/2(Time)
  If/2 -> If Action Subsystem1/Action
  If/1 -> If Action Subsystem/Action

== system BESS_Harness/BESS/Detailed/BESS Controller/Grid Forming/Measurement/abc2dq/Supply Current to dq ==
  abc : Inport
  Angle : Inport  Port=2
  Demux : Demux  Outputs=3
  Park Transform : eeTransforms/Park Transform  AxisAlignment=D-axis  PowerInvariant=off
  Terminator : Terminator
  Igd : Outport  VectorParamsAs1DForOutWhenUnconnected=off
  Igq : Outport  Port=2  VectorParamsAs1DForOutWhenUnconnected=off
  wires:
  Angle/1 -> Park Transform/2
  abc/1 -> Park Transform/1
  Demux/1 -> Igd/1
  Demux/2 -> Igq/1
  Park Transform/1 -> Demux/1
  Demux/3 -> Terminator/1

== system BESS_Harness/BESS/Detailed/BESS Controller/Grid Forming/Measurement/abc2dq/Supply Voltage  to dq1 ==
  Angle : Inport
  abc : Inport  Port=2
  Demux : Demux  Outputs=3
  Park Transform : eeTransforms/Park Transform  AxisAlignment=D-axis  PowerInvariant=off
  Terminator : Terminator
  Vgd : Outport  VectorParamsAs1DForOutWhenUnconnected=off
  Vgq : Outport  Port=2  VectorParamsAs1DForOutWhenUnconnected=off
  wires:
  Angle/1 -> Park Transform/2
  abc/1 -> Park Transform/1
  Demux/1 -> Vgd/1
  Demux/2 -> Vgq/1
  Park Transform/1 -> Demux/1
  Demux/3 -> Terminator/1

== system BESS_Harness/BESS/Detailed/BESS Controller/Grid Forming/Power Control/ActivePowerControl/droopControl ==
  Pref : Inport
  Pmeas : Inport  Port=2
  fref : Inport  Port=3
  cntrlflag : Inport  Port=4
  fgrid : Inport  Port=5
  Add : Sum  Inputs=+-
  Constant : Constant
  Constant5 : Constant  Value=pi/2
  Gain : Gain  Gain=powerFreq*2*pi
  Integrator with Wrapped State (Discrete or Continuous) : eeGeneralControl/Integrator with Wrapped State (Discrete or Continuous)  LabelModeActiveChoice=Discrete  WrappedStateUpperValue=2*pi  WrappedStateLowerValue=0  x0=0  Ts=activePowerSampleTime
  Lead-Lag (Discrete or Continuous) : eeGeneralControl/Lead-Lag (Discrete or Continuous)  T1=droopT1  T2=droopT2  B=inf  A=-inf  init_option=Inherited from block input  x0=0  Ts=activePowerSampleTime
  Low-Pass Filter (Discrete or Continuous) : eeGeneralControl/Low-Pass Filter (Discrete or Continuous)  K=1  T=droopTC  B=inf  A=-inf  init_option=Specify as parameter  x0=0  Ts=activePowerSampleTime
  Scope : Scope
  Scope1 : Scope
  Scope2 : Scope
  Sum : Sum  Inputs=|-+
  Sum1 : Sum  Inputs=|-+
  Terminator : Terminator
  Terminator1 : Terminator
  Terminator2 : Terminator
  mp : Gain  Gain=droopSlope
  Theta : Outport
  w : Outport  Port=2
  wires:
  cntrlflag/1 -> Terminator2/1
  fref/1 -> Terminator1/1
  fgrid/1 -> Terminator/1
  Sum1/1 -> Gain/1
  Constant/1 -> Sum1/2
  Integrator with Wrapped State (Discrete or Continuous)/1 -> Add/1
  Lead-Lag (Discrete or Continuous)/1 -> Sum/2
  Gain/1 -> w/1, Integrator with Wrapped State (Discrete or Continuous)/1
  Pref/1 -> Sum/1
  Constant5/1 -> Add/2
  Add/1 -> Theta/1, Scope1/1
  Pmeas/1 -> Lead-Lag (Discrete or Continuous)/1
  Sum/1 -> mp/1, Scope/1
  mp/1 -> Low-Pass Filter (Discrete or Continuous)/1
  Low-Pass Filter (Discrete or Continuous)/1 -> Sum1/1, Scope2/1

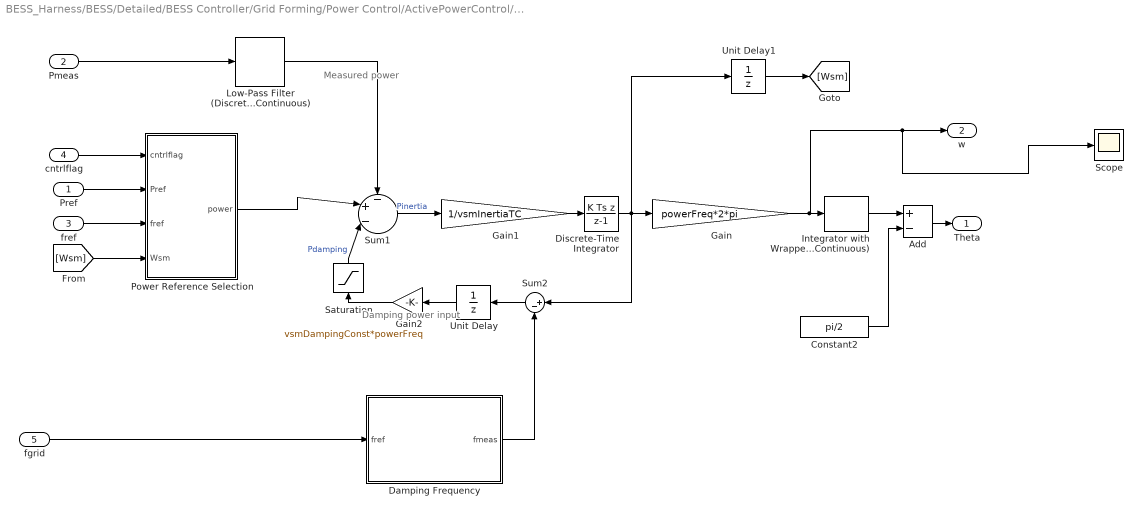
== system BESS_Harness/BESS/Detailed/BESS Controller/Grid Forming/Power Control/ActivePowerControl/vsmControl ==
  note: Damping power input
  note: Measured power
  Pref : Inport
  Pmeas : Inport  Port=2
  fref : Inport  Port=3
  cntrlflag : Inport  Port=4
  fgrid : Inport  Port=5
  Add : Sum  Inputs=+-
  Constant2 : Constant  Value=pi/2
  Damping Frequency : Subsystem  Variant=on  VariantControlMode=label  VariantControl=Choice  LabelModeActiveChoice=constFreq
  Discrete-Time Integrator : DiscreteIntegrator  IntegratorMethod=Integration: Backward Euler  InitialCondition=1  SampleTime=activePowerSampleTime  LimitOutput=on  UpperSaturationLimit=1.1  LowerSaturationLimit=0.9  ICPrevOutput=DiscIntNeverNeededParam  ICPrevScaledInput=DiscIntNeverNeededParam
  Gain : Gain  Gain=powerFreq*2*pi
  Gain1 : Gain  Gain=1/vsmInertiaTC
  Gain2 : Gain  Gain=vsmDampingConst*powerFreq
  Integrator with Wrapped State (Discrete or Continuous) : eeGeneralControl/Integrator with Wrapped State (Discrete or Continuous)  LabelModeActiveChoice=Discrete  WrappedStateUpperValue=2*pi  WrappedStateLowerValue=0  x0=0  Ts=activePowerSampleTime
  Low-Pass Filter (Discrete or Continuous) : eeGeneralControl/Low-Pass Filter (Discrete or Continuous)  K=1  T=vsmPmeasFilterTC  B=inf  A=-inf  init_option=Specify as parameter  x0=0  Ts=activePowerSampleTime
  Power Reference Selection : Subsystem
  Saturation : Saturate  UpperLimit=dampingPowerMaxLimit  LowerLimit=dampingPowerMinLimit
  Scope : Scope
  Sum1 : Sum  Inputs=-+-|
  Sum2 : Sum  Inputs=|+-
  Unit Delay : UnitDelay  SampleTime=-1  HasFrameUpgradeWarning=on
  Unit Delay1 : UnitDelay  SampleTime=-1  HasFrameUpgradeWarning=on
  Theta : Outport
  w : Outport  Port=2
  wires:
  [Wsm] -> Power Reference Selection/4(Wsm)
  Pmeas/1 -> Low-Pass Filter (Discrete or Continuous)/1
  fref/1 -> Power Reference Selection/3(fref)
  Pref/1 -> Power Reference Selection/2(Pref)
  cntrlflag/1 -> Power Reference Selection/1(cntrlflag)
  Damping Frequency/1(fmeas) -> Sum2/2
  fgrid/1 -> Damping Frequency/1(fref)
  Saturation/1 -> Sum1/3  "Pdamping"
  Unit Delay1/1 -> [Wsm]
  Unit Delay/1 -> Gain2/1
  Gain/1 -> w/1, Scope/1, Integrator with Wrapped State (Discrete or Continuous)/1
  Gain1/1 -> Discrete-Time Integrator/1
  Sum2/1 -> Unit Delay/1
  Power Reference Selection/1(power) -> Sum1/2
  Gain2/1 -> Saturation/1
  Low-Pass Filter (Discrete or Continuous)/1 -> Sum1/1
  Discrete-Time Integrator/1 -> Sum2/1, Unit Delay1/1, Gain/1
  Add/1 -> Theta/1
  Constant2/1 -> Add/2
  Sum1/1 -> Gain1/1  "Pinertia"
  Integrator with Wrapped State (Discrete or Continuous)/1 -> Add/1

== system BESS_Harness/BESS/Detailed/BESS Controller/Grid Forming/Power Control/ReactiveControl/Voltage  Reference Selection ==
  cntrlflag : Inport
  Qref : Inport  Port=2
  Qmeas : Inport  Port=3
  Vref : Inport  Port=4
  Vgdmeas : Inport  Port=5
  If : If
  If Action Subsystem : Subsystem  TreatAsAtomicUnit=on
  If Action Subsystem1 : Subsystem  TreatAsAtomicUnit=on
  Merge : Merge
  Rate Transition : RateTransition
  Vd : Outport
  wires:
  Rate Transition/1 -> If/1
  Vgdmeas/1 -> If Action Subsystem1/2(Vmeas)
  Vref/1 -> If Action Subsystem1/1(Vref)
  If Action Subsystem1/1(Voltage) -> Merge/2
  Qref/1 -> If Action Subsystem/1(Qref)
  Qmeas/1 -> If Action Subsystem/2(Qmeas)
  Merge/1 -> Vd/1
  cntrlflag/1 -> Rate Transition/1
  If/2 -> If Action Subsystem1/Action
  If Action Subsystem/1(Vd) -> Merge/1
  If/1 -> If Action Subsystem/Action

== system BESS_Harness/BESS/Detailed/BESS Controller/Grid Forming/VoltageCurrentControl/Controller/Id Current Limiting ==
  Imax : Inport
  Id : Inport  Port=2
  Abs : Abs  SaturateOnIntegerOverflow=off
  Switch : Switch  Criteria=u2 > Threshold  SaturateOnIntegerOverflow=off  InputSameDT=off
  Idref : Outport
  wires:
  Switch/1 -> Idref/1
  Imax/1 -> Switch/1, Abs/1
  Abs/1 -> Switch/2
  Id/1 -> Switch/3

== system BESS_Harness/BESS/Detailed/BESS Controller/Grid Forming/VoltageCurrentControl/Controller/Iq Current Limiting ==
  Imax : Inport
  Iq : Inport  Port=2
  Abs : Abs  SaturateOnIntegerOverflow=off
  Switch : Switch  Criteria=u2 > Threshold  SaturateOnIntegerOverflow=off  InputSameDT=off
  Iqref : Outport
  wires:
  Switch/1 -> Iqref/1
  Imax/1 -> Switch/1, Abs/1
  Abs/1 -> Switch/2
  Iq/1 -> Switch/3

== system BESS_Harness/BESS/Detailed/BESS Controller/Grid Forming/VoltageCurrentControl/Controller/Voltage control ==
  e : Inport
  resetBlackStart : Inport  Port=2
  Discrete-Time Integrator : DiscreteIntegrator  IntegratorMethod=Integration: Backward Euler  ExternalReset=level  SampleTime=voltControlTs  LimitOutput=on  UpperSaturationLimit=VdMaxCt  LowerSaturationLimit=VdMinCt  ICPrevOutput=DiscIntNeverNeededParam  ICPrevScaledInput=DiscIntNeverNeededParam
  Ki : Gain  Gain=VdIGain
  Kp : Gain  Gain=vdPGain
  Limit : Saturate  UpperLimit=VdMaxCt  LowerLimit=VdMinCt
  Scope : Scope  NumInputPorts=2
      settings: ActiveDisplayYMinimum=-2.29888  ActiveDisplayYMaximum=11.36654  DataLoggingVariableName=ScopeData7
  Scope1 : Scope
      settings: ActiveDisplayYMinimum=-0.22989  ActiveDisplayYMaximum=1.13665  DataLoggingVariableName=ScopeData8
  Sum7 : Sum  Inputs=|++
  u : Outport  VectorParamsAs1DForOutWhenUnconnected=off
  wires:
  resetBlackStart/1 -> Discrete-Time Integrator/2
  e/1 -> Scope1/1, Ki/1, Kp/1
  Sum7/1 -> Limit/1
  Ki/1 -> Discrete-Time Integrator/1
  Limit/1 -> u/1
  Kp/1 -> Scope/1, Sum7/1
  Discrete-Time Integrator/1 -> Scope/2, Sum7/2

== system BESS_Harness/BESS/Detailed/BESS Controller/Grid Forming/VoltageCurrentControl/Controller/Voltage control1 ==
  e : Inport
  resetBlackStart : Inport  Port=2
  Discrete-Time Integrator : DiscreteIntegrator  IntegratorMethod=Integration: Backward Euler  ExternalReset=level  SampleTime=voltControlTs  LimitOutput=on  UpperSaturationLimit=VqMaxCt  LowerSaturationLimit=VqMinCt  ICPrevOutput=DiscIntNeverNeededParam  ICPrevScaledInput=DiscIntNeverNeededParam
  Ki : Gain  Gain=VqIGain
  Kp : Gain  Gain=VqPGain
  Limit : Saturate  UpperLimit=VqMaxCt  LowerLimit=VqMinCt
  Sum7 : Sum  Inputs=|++
  u : Outport  VectorParamsAs1DForOutWhenUnconnected=off
  wires:
  resetBlackStart/1 -> Discrete-Time Integrator/2
  Limit/1 -> u/1
  Ki/1 -> Discrete-Time Integrator/1
  Kp/1 -> Sum7/1
  e/1 -> Kp/1, Ki/1
  Sum7/1 -> Limit/1
  Discrete-Time Integrator/1 -> Sum7/2

== system BESS_Harness/BESS/Detailed/BESS Controller/Grid Forming/VoltageCurrentControl/Controller/d-axis current control ==
  e : Inport
  resetBlackStart : Inport  Port=2
  Discrete-Time Integrator : DiscreteIntegrator  IntegratorMethod=Integration: Backward Euler  ExternalReset=level  SampleTime=currentControlTs  LimitOutput=on  UpperSaturationLimit=4  LowerSaturationLimit=-4  ICPrevOutput=DiscIntNeverNeededParam  ICPrevScaledInput=DiscIntNeverNeededParam
  Ki : Gain  Gain=IdIGain
  Kp : Gain  Gain=IdPGain
  Limit : Saturate  UpperLimit=4  LowerLimit=-4
  Sum7 : Sum  Inputs=|++
  u : Outport  VectorParamsAs1DForOutWhenUnconnected=off
  wires:
  resetBlackStart/1 -> Discrete-Time Integrator/2
  Ki/1 -> Discrete-Time Integrator/1
  Limit/1 -> u/1
  Kp/1 -> Sum7/1
  e/1 -> Kp/1, Ki/1
  Sum7/1 -> Limit/1
  Discrete-Time Integrator/1 -> Sum7/2

== system BESS_Harness/BESS/Detailed/BESS Controller/Grid Forming/VoltageCurrentControl/Controller/q-axis current control ==
  e : Inport
  resetBlackStart : Inport  Port=2
  Discrete-Time Integrator : DiscreteIntegrator  IntegratorMethod=Integration: Backward Euler  ExternalReset=level  SampleTime=currentControlTs  LimitOutput=on  UpperSaturationLimit=3  LowerSaturationLimit=-3  ICPrevOutput=DiscIntNeverNeededParam  ICPrevScaledInput=DiscIntNeverNeededParam
  Ki : Gain  Gain=IqIGain
  Kp : Gain  Gain=IqPGain
  Limit : Saturate  UpperLimit=3  LowerLimit=-3
  Sum7 : Sum  Inputs=|++
  u : Outport  VectorParamsAs1DForOutWhenUnconnected=off
  wires:
  resetBlackStart/1 -> Discrete-Time Integrator/2
  Discrete-Time Integrator/1 -> Sum7/2
  Limit/1 -> u/1
  Sum7/1 -> Limit/1
  e/1 -> Ki/1, Kp/1
  Kp/1 -> Sum7/1
  Ki/1 -> Discrete-Time Integrator/1

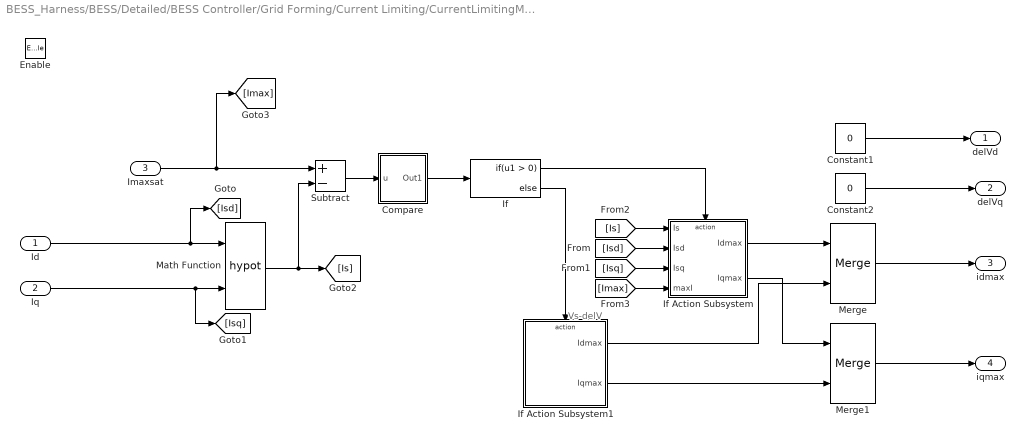
== system BESS_Harness/BESS/Detailed/BESS Controller/Grid Forming/Current Limiting/CurrentLimitingMethod/currentLimitAndVirtual/Current Saturation ==
  note: Vs-delV
  Id : Inport
  Iq : Inport  Port=2
  Imaxsat : Inport  Port=3
  Enable : EnablePort
  Compare : Subsystem
  Constant1 : Constant  Value=0
  Constant2 : Constant  Value=0
  If : If
  If Action Subsystem : Subsystem  TreatAsAtomicUnit=on
  If Action Subsystem1 : Subsystem  TreatAsAtomicUnit=on
  Math Function : Math  Operator=hypot
  Merge : Merge
  Merge1 : Merge
  Subtract : Sum  Inputs=+-
  delVd : Outport
  delVq : Outport  Port=2
  idmax : Outport  Port=3
  iqmax : Outport  Port=4
  wires:
  [Imax] -> If Action Subsystem/4(maxI)
  Imaxsat/1 -> Subtract/1, [Imax]
  Merge1/1 -> iqmax/1
  [Isq] -> If Action Subsystem/3(Isq)
  Constant1/1 -> delVd/1
  [Isd] -> If Action Subsystem/2(Isd)
  Merge/1 -> idmax/1
  If Action Subsystem1/2(Iqmax) -> Merge1/2
  Id/1 -> Math Function/1, [Isd]
  [Is] -> If Action Subsystem/1(Is)
  If Action Subsystem/1(Idmax) -> Merge/1
  Compare/1(Out1) -> If/1
  Subtract/1 -> Compare/1(u)
  If Action Subsystem/2(Iqmax) -> Merge1/1
  If/2 -> If Action Subsystem1/Action
  Math Function/1 -> Subtract/2, [Is]
  Constant2/1 -> delVq/1
  If Action Subsystem1/1(Idmax) -> Merge/2
  If/1 -> If Action Subsystem/Action
  Iq/1 -> Math Function/2, [Isq]

== system BESS_Harness/BESS/Detailed/BESS Controller/Grid Forming/Current Limiting/CurrentLimitingMethod/currentLimitAndVirtual/No Fault Ride Through ==
  Id : Inport
  Iq : Inport  Port=2
  Enable : EnablePort
  Constant{1..4} (4 alike) : Constant  Value=0
  Terminator : Terminator
  Terminator1 : Terminator
  delVd : Outport
  delVq : Outport  Port=2
  idmax : Outport  Port=3
  iqmax : Outport  Port=4
  wires:
  Iq/1 -> Terminator1/1
  Id/1 -> Terminator/1
  Constant4/1 -> delVq/1
  Constant1/1 -> delVd/1
  Constant2/1 -> idmax/1
  Constant3/1 -> iqmax/1

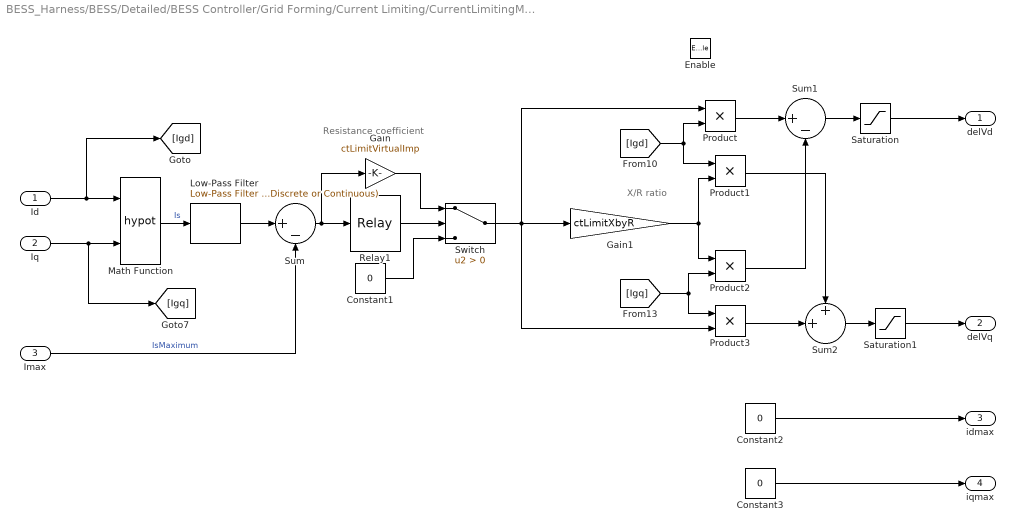
== system BESS_Harness/BESS/Detailed/BESS Controller/Grid Forming/Current Limiting/CurrentLimitingMethod/currentLimitAndVirtual/VI ==
  note: X/R ratio
  note: Resistance coefficient
  Id : Inport
  Iq : Inport  Port=2
  Imax : Inport  Port=3
  Enable : EnablePort
  Constant1 : Constant  Value=0
  Constant2 : Constant  Value=0
  Constant3 : Constant  Value=0
  Gain : Gain  Gain=ctLimitVirtualImp
  Gain1 : Gain  Gain=ctLimitXbyR
  Low-Pass Filter : eeGeneralControl/Low-Pass Filter (Discrete or Continuous)  K=1  T=currentVITimeConst  B=inf  A=-inf  init_option=Inherited from block input  x0=0  Ts=-1
  Math Function : Math  Operator=hypot
  Product{,1..3} (4 alike) : Product
  Relay1 : Relay  OnSwitchValue=0.01  OffSwitchValue=-0.1
  Saturation : Saturate  UpperLimit=1  LowerLimit=-1
  Saturation1 : Saturate  UpperLimit=1  LowerLimit=-1
  Sum : Sum  Inputs=|+-
  Sum1 : Sum  Inputs=|+-
  Sum2 : Sum  Inputs=++|
  Switch : Switch  Criteria=u2 > Threshold  SaturateOnIntegerOverflow=off  InputSameDT=off
  delVd : Outport
  delVq : Outport  Port=2
  idmax : Outport  Port=3
  iqmax : Outport  Port=4
  wires:
  Imax/1 -> Sum/2  "IsMaximum"
  Low-Pass Filter/1 -> Sum/1
  Relay1/1 -> Switch/2
  Constant2/1 -> idmax/1
  Constant3/1 -> iqmax/1
  Saturation/1 -> delVd/1
  Constant1/1 -> Switch/3
  Gain/1 -> Switch/1
  Product2/1 -> Sum1/2
  Product1/1 -> Sum2/1
  Saturation1/1 -> delVq/1
  [Igd] -> Product/2, Product1/1
  Switch/1 -> Gain1/1, Product/1, Product3/2
  Math Function/1 -> Low-Pass Filter/1  "Is"
  Iq/1 -> Math Function/2, [Igq]
  [Igq] -> Product2/2, Product3/1
  Product/1 -> Sum1/1
  Sum1/1 -> Saturation/1
  Sum/1 -> Relay1/1, Gain/1
  Sum2/1 -> Saturation1/1
  Id/1 -> [Igd], Math Function/1
  Product3/1 -> Sum2/2
  Gain1/1 -> Product2/1, Product1/2
